simulink model "classical_control"  (R2023a)
settings: Solver=VariableStepAuto  StartTime=0.0  StopTime=20  RelTol=1e-10
settings Model: Creator=ganes  LastModifiedBy=ganes

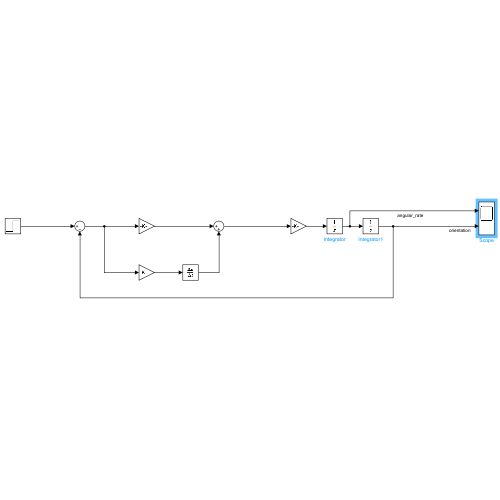
[thumbnail: Simulink's stored preview of the top-level diagram]
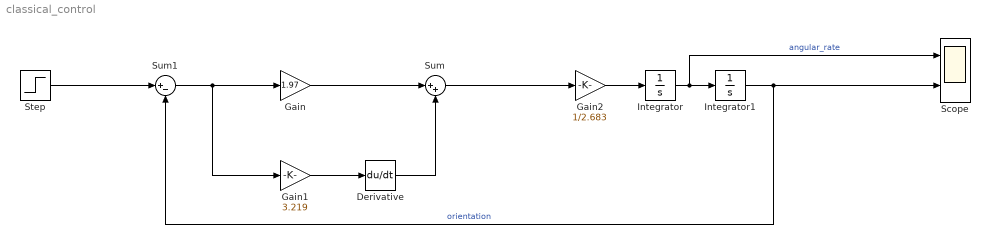
== system classical_control ==
  Derivative : Derivative
  Gain : Gain  Gain=1.97
  Gain1 : Gain  Gain=3.219
  Gain2 : Gain  Gain=1/2.683
  Integrator : Integrator
  Integrator1 : Integrator
  Scope : Scope  NumInputPorts=2
  Step : Step  Time=0  SampleTime=0
  Sum : Sum  Inputs=|++
  Sum1 : Sum  Inputs=|+-
  wires:
  Step/1 -> Sum1/1
  Sum1/1 -> Gain1/1, Gain/1
  Gain/1 -> Sum/1
  Sum/1 -> Gain2/1
  Gain2/1 -> Integrator/1
  Integrator/1 -> Scope/1, Integrator1/1  "angular_rate"
  Integrator1/1 -> Scope/2, Sum1/2  "orientation"
  Gain1/1 -> Derivative/1
  Derivative/1 -> Sum/2
